simulink model "lqr_robot"  (R2020b)
settings: Solver=VariableStepAuto  StartTime=0.0  StopTime=10.0  RelTol=1e-3
values from neighbouring files (symbols this model uses):
  g = 9.81    [kalman_jacobian.m]    (also in parametriEgo.m = [0; 0; -9.81])
  initial_conditions = [0,0,0*pi/180,0*pi/180,0,0]    [parametriEgo.m]
  L = 0.379    [parametriEgo.m]
  l = 0.248    [parametriEgo.m]
  mb = 21.7+0.536*10+0.381*2    (= 27.822)    [parametriEgo.m]
  mw = 1.6    [parametriEgo.m]
  r = 0.13    [parametriEgo.m]
  tau_max = 11    [parametriEgo.m]
  TsGraph = 1/100    (= 0.01)    [parametriEgo.m]
undefined symbols (not defined in the file or in its folder): alpha
settings Model: Creator=stefa  LastModifiedBy=stefa

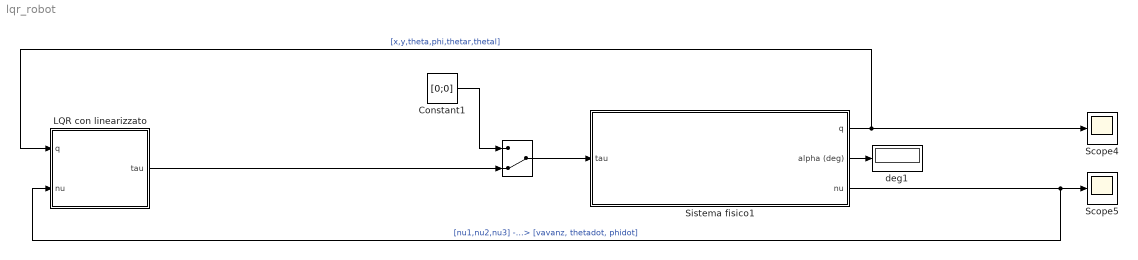
== system lqr_robot ==
  " " : ManualSwitch  CurrentSetting=0
  Constant1 : Constant  Value=[0;0]
  LQR con linearizzato : Subsystem
  Scope4 : Scope
  Scope5 : Scope
  Sistema fisico1 : Subsystem
  deg1 : Display
  wires:
  Constant1/1 -> " "/1
  " "/1 -> Sistema fisico1/1(tau)
  Sistema fisico1/1(q) -> LQR con linearizzato/1(q), Scope4/1  "[x,y,theta,phi,thetar,thetal]"
  Sistema fisico1/2(alpha (deg)) -> deg1/1
  LQR con linearizzato/1(tau) -> " "/2
  Sistema fisico1/3(nu) -> LQR con linearizzato/2(nu), Scope5/1  "[nu1,nu2,nu3] -> [vavanz, thetadot, phidot]"

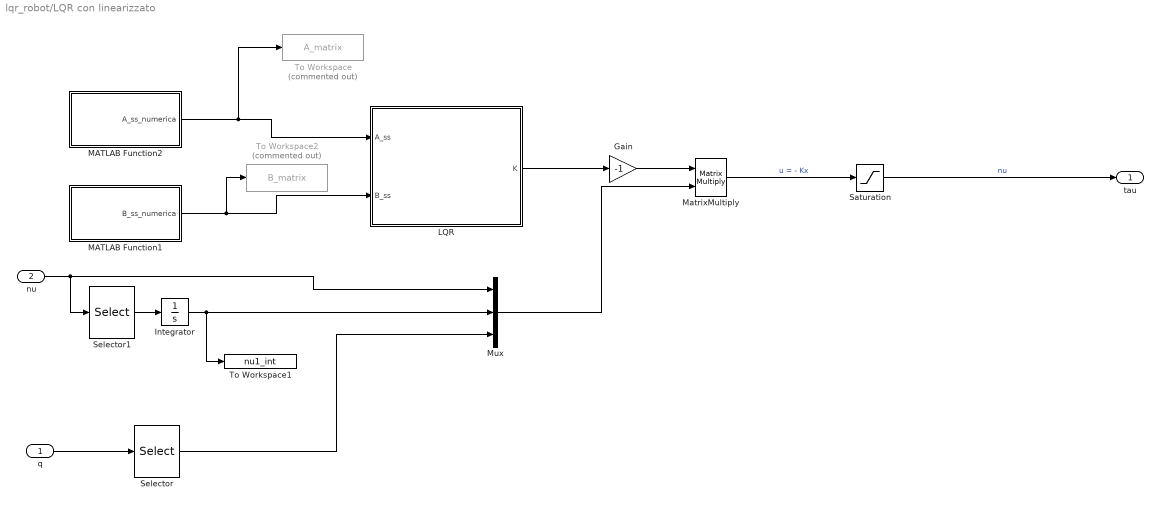
== system lqr_robot/LQR con linearizzato ==
  q : Inport
  nu : Inport  Port=2
  Gain : Gain  Gain=-1
  Integrator : Integrator
  LQR : MATLAB Function  TreatAsAtomicUnit=on
  MATLAB Function1 : MATLAB Function  TreatAsAtomicUnit=on
  MATLAB Function2 : MATLAB Function  TreatAsAtomicUnit=on
  MatrixMultiply : Product  Multiplication=Matrix(*)
  Mux : Mux  Inputs=3
  Saturation : Saturate  UpperLimit=tau_max  LowerLimit=-tau_max
  Selector : Selector  InputPortWidth=6  IndexOptions=Index vector (dialog)  Indices=[3 4]  OutputSizes=1
  Selector1 : Selector  InputPortWidth=3  IndexOptions=Index vector (dialog)  Indices=1  OutputSizes=1
  To Workspace : ToWorkspace  Commented=on  VariableName=A_matrix  SampleTime=-1
      settings: MaxDataPoints=1
  To Workspace1 : ToWorkspace  VariableName=nu1_int  SaveFormat=Timeseries  SampleTime=TsGraph
  To Workspace2 : ToWorkspace  Commented=on  VariableName=B_matrix  SampleTime=-1
      settings: MaxDataPoints=1
  tau : Outport
  wires:
  MATLAB Function1/1(B_ss_numerica) -> To Workspace2/1, LQR/2(B_ss)
  LQR/1(K) -> Gain/1
  MATLAB Function2/1(A_ss_numerica) -> To Workspace/1, LQR/1(A_ss)
  Gain/1 -> MatrixMultiply/1
  MatrixMultiply/1 -> Saturation/1  "u = - Kx"
  nu/1 -> Selector1/1, Mux/1
  q/1 -> Selector/1
  Mux/1 -> MatrixMultiply/2
  Selector/1 -> Mux/3
  Saturation/1 -> tau/1  "nu"
  Selector1/1 -> Integrator/1
  Integrator/1 -> Mux/2, To Workspace1/1

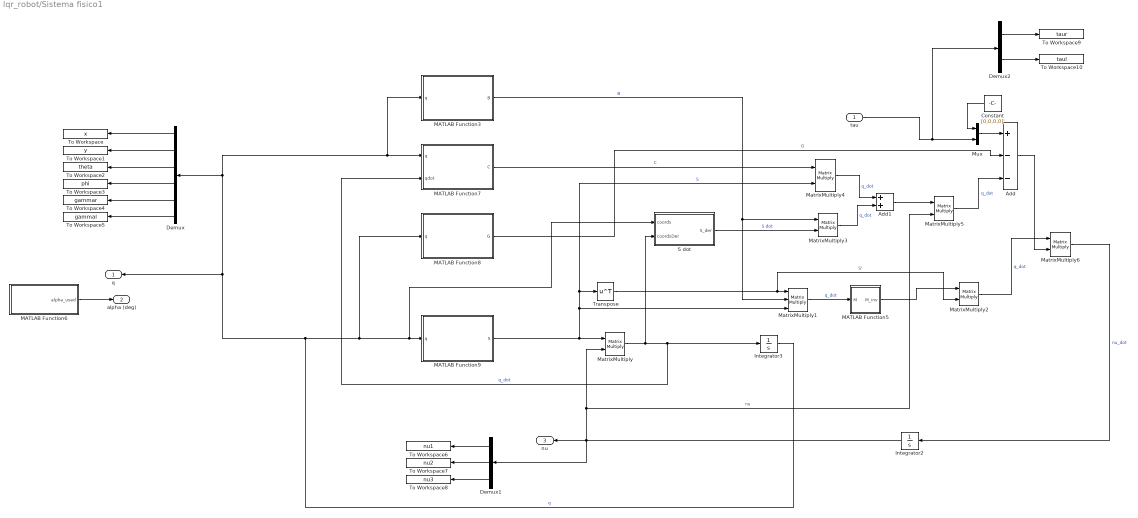
== system lqr_robot/Sistema fisico1 ==
  tau : Inport
  Add : Sum  Inputs=+--
  Add1 : Sum
  Constant : Constant  Value=[0,0,0,0]'
  Demux : Demux  Outputs=6
  Demux1 : Demux  Outputs=3
  Demux2 : Demux  Outputs=2
  Integrator2 : Integrator  InitialCondition=[0; 0; 0]
  Integrator3 : Integrator  InitialCondition=initial_conditions
  MATLAB Function3 : MATLAB Function  TreatAsAtomicUnit=on
  MATLAB Function5 : MATLAB Function  TreatAsAtomicUnit=on
  MATLAB Function6 : MATLAB Function  TreatAsAtomicUnit=on
  MATLAB Function7 : MATLAB Function  TreatAsAtomicUnit=on
  MATLAB Function8 : MATLAB Function  TreatAsAtomicUnit=on
  MATLAB Function9 : MATLAB Function  TreatAsAtomicUnit=on
  MatrixMultiply{,2..6} (6 alike) : Product  Multiplication=Matrix(*)
  MatrixMultiply1 : Product  Inputs=3  Multiplication=Matrix(*)
  Mux : Mux  Inputs=2
  S dot : MATLAB Function  TreatAsAtomicUnit=on
  To Workspace : ToWorkspace  VariableName=x  SaveFormat=Timeseries  SampleTime=TsGraph
  To Workspace1 : ToWorkspace  VariableName=y  SaveFormat=Timeseries  SampleTime=TsGraph
  To Workspace10 : ToWorkspace  VariableName=taul  SaveFormat=Timeseries  SampleTime=TsGraph
  To Workspace2 : ToWorkspace  VariableName=theta  SaveFormat=Timeseries  SampleTime=TsGraph
  To Workspace3 : ToWorkspace  VariableName=phi  SaveFormat=Timeseries  SampleTime=TsGraph
  To Workspace4 : ToWorkspace  VariableName=gammar  SaveFormat=Timeseries  SampleTime=TsGraph
  To Workspace5 : ToWorkspace  VariableName=gammal  SaveFormat=Timeseries  SampleTime=TsGraph
  To Workspace6 : ToWorkspace  VariableName=nu1  SaveFormat=Timeseries  SampleTime=TsGraph
  To Workspace7 : ToWorkspace  VariableName=nu2  SaveFormat=Timeseries  SampleTime=TsGraph
  To Workspace8 : ToWorkspace  VariableName=nu3  SaveFormat=Timeseries  SampleTime=TsGraph
  To Workspace9 : ToWorkspace  VariableName=taur  SaveFormat=Timeseries  SampleTime=TsGraph
  Transpose : Math  Operator=transpose  SaturateOnIntegerOverflow=on
  q : Outport
  alpha (deg) : Outport  Port=2
  nu : Outport  Port=3
  wires:
  MATLAB Function9/1(S) -> MatrixMultiply1/3, Transpose/1, MatrixMultiply4/2, MatrixMultiply/1  "S"
  Integrator3/1 -> MATLAB Function3/1(q), MATLAB Function7/1(q), Demux/1, q/1, MATLAB Function8/1(q), MATLAB Function9/1(q), S dot/1(coords)  "q"
  S dot/1(S_der) -> MatrixMultiply3/2  "S dot"
  MATLAB Function3/1(B) -> MatrixMultiply3/1, MatrixMultiply1/2  "B"
  Integrator2/1 -> Demux1/1, MatrixMultiply5/2, MatrixMultiply/2, nu/1  "nu"
  MATLAB Function8/1(G) -> Add/2  "G"
  Transpose/1 -> MatrixMultiply2/2, MatrixMultiply1/1  "S'"
  MatrixMultiply1/1 -> MATLAB Function5/1(M)  "q_dot"
  MatrixMultiply3/1 -> Add1/2  "q_dot"
  MatrixMultiply/1 -> MATLAB Function7/2(qdot), Integrator3/1, S dot/2(coordsDer)  "q_dot"
  MATLAB Function7/1(C) -> MatrixMultiply4/1  "C"
  Add1/1 -> MatrixMultiply5/1
  MatrixMultiply4/1 -> Add1/1  "q_dot"
  MatrixMultiply5/1 -> Add/3  "q_dot"
  Add/1 -> MatrixMultiply6/2
  MatrixMultiply6/1 -> Integrator2/1  "nu_dot"
  MATLAB Function5/1(M_inv) -> MatrixMultiply2/1
  MatrixMultiply2/1 -> MatrixMultiply6/1  "q_dot"
  MATLAB Function6/1(alpha_used) -> alpha (deg)/1
  Demux/5 -> To Workspace4/1
  Demux/2 -> To Workspace1/1
  Demux/1 -> To Workspace/1
  Demux/3 -> To Workspace2/1
  Demux/4 -> To Workspace3/1
  Demux/6 -> To Workspace5/1
  Mux/1 -> Add/1
  Constant/1 -> Mux/1
  Demux1/1 -> To Workspace6/1
  Demux1/2 -> To Workspace7/1
  Demux1/3 -> To Workspace8/1
  tau/1 -> Demux2/1, Mux/2
  Demux2/1 -> To Workspace9/1
  Demux2/2 -> To Workspace10/1

== matlab function lqr_robot/LQR con linearizzato/LQR ==
  data: A_ss input; K output; B_ss input
function K = fcn(A_ss, B_ss)

Q = eye(6);
R = eye(2);

% state: nu1, nu2, nu3, nu1_int, theta, phi

Q = [500,0,0,0,0,0;
    0,10,0,0,0,0;
    0,0,10,0,0,0;
    0,0,0,10000,0,0;
    0,0,0,0,100,0;
    0,0,0,0,0,400];

R = [0.1,0;
    0,0.1];

coder.extrinsic('lqr')

K = zeros(2, 6);

K = lqr(A_ss, B_ss, Q, R);
end

== matlab function lqr_robot/LQR con linearizzato/MATLAB Function1 ==
  data: B_ss_numerica output
function B_ss_numerica = B_ss_num()

%theta= pi/2;
theta= 0;
phi = 0;
%phi = -alpha;

B_ss_numerica=B_ss_file(phi,theta);

== matlab function lqr_robot/LQR con linearizzato/MATLAB Function2 ==
  data: A_ss_numerica output
function A_ss_numerica = A_ss_num()

%theta= pi/2;
theta= 0;
%phi = -alpha;
phi = 0;

thetadot = 0;
phidot = 0;

nu1 = 0;
nu2 = 0;
nu3 = 0;
taul=0;
taur=0;

A_ss_numerica=A_ss_file(alpha,nu1,nu2,nu3,phi,taul,taur,theta);

== matlab function lqr_robot/Sistema fisico1/MATLAB Function5 ==
  data: M input; M_inv output
function M_inv = inverse(M)

M_inv = inv(M);

== matlab function lqr_robot/Sistema fisico1/MATLAB Function6 ==
  data: alpha_used output; alpha parameter
function alpha_used = from_workspace(alpha)

alpha_used=alpha*180/pi;

== matlab function lqr_robot/Sistema fisico1/S dot ==
  data: coords input; S_der output; r parameter; coordsDer input
function S_der = matrix_S_der(coords,r, coordsDer)

theta = coords(3);
thetadot = coordsDer(3);

S_der = zeros(6,3);

S_der = [-cos(theta)*thetadot, 0, 0;
    -sin(theta)*thetadot, 0, 0;
    0, 0, 0;
    0, 0, 0;
    0, 0, 0;
    0, 0, 0];

== matlab function lqr_robot/Sistema fisico1/MATLAB Function3 ==
  data: q input; B output; alpha parameter
function B = matrix_B(q, alpha)
theta = q(3);
phi = q(4);

B=B_dynamic_matrix(phi, theta);

== matlab function lqr_robot/Sistema fisico1/MATLAB Function7 ==
  data: q input; qdot input; C output; alpha parameter
function C = matrix_C(q, qdot, alpha)
theta = q(3);
phi = q(4);

thetadot = qdot(3);
phidot = qdot(4);

C=C_dynamic_matrix(phi,phidot,theta,thetadot);

== matlab function lqr_robot/Sistema fisico1/MATLAB Function8 ==
  data: q input; G output; mw parameter; mb parameter; g parameter; alpha parameter; L parameter
function G = vector_G(q, mw, mb, g, alpha, L)

theta = q(3);
phi = q(4);

G = G_dynamic_vector(alpha,phi,theta)

== matlab function lqr_robot/Sistema fisico1/MATLAB Function9 ==
  data: q input; S output; r parameter; l parameter
function S = matrix_S(q, r, l)
theta = q(3);

S = [-sin(theta), 0, 0;
    cos(theta), 0, 0;
    0, 1, 0;
    0, 0, 1;
    -1/r, -l/r, -1;
    -1/r, l/r, -1];
